simulink model "Quad_Nonlinear_Pitch_PID"  (R2020a)
settings: Solver=ode4  StartTime=0.0  StopTime=15  FixedStep=0.01  RelTol=1e-3
InitFcn:
  | QuadParameter
values from neighbouring files (symbols this model uses):
  AHRS_RCP = AHRS(251:end, :) * pi / 180    [PS_II.m]    (also in RCP_data_I.m; RCP_data_II.m)
  b = 3.13e-5    (= 3.13e-05)    [QuadParameter.m]
  d_cg = 0.2    [QuadParameter.m]
  g = 9.81    [QuadParameter.m]
  h_cg = 0.02    [QuadParameter.m]
  J_yy = 0.03066    [QuadParameter.m]
  KD_Pitch = 10^savedata{1}(3)/15    [RCP_data_I.m]    (also in RCP_data_II.m)
  KI_Pitch = 10^savedata{1}(2)*10    [RCP_data_I.m]    (also in RCP_data_II.m)
  KP_Pitch = 10^savedata{1}(1)/25    [RCP_data_I.m]    (also in RCP_data_II.m)
  m_tot = 0.638    [QuadParameter.m]
undefined symbols (not defined in the file or in its folder): m2, magnitude, miu_k, r_y
libraries: simulink x1
settings Model: OrderedModelArguments=off  Creator=Ali  LastModifiedBy=Ali

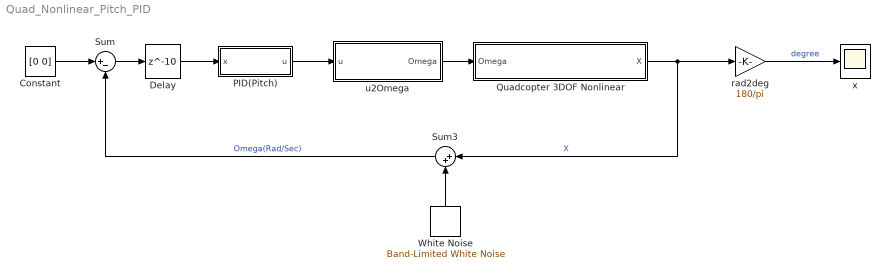
== system Quad_Nonlinear_Pitch_PID ==
  " White Noise" : simulink/Sources/Band-Limited White Noise  Cov=[0.000005]  Ts=.01  seed=[23341]
  Constant : Constant  Value=[0 0]
  Delay : Delay  DelayLength=10
  PID(Pitch) : Subsystem
  Quadcopter 3DOF Nonlinear : Subsystem  TreatAsAtomicUnit=on
  Sum : Sum  Inputs=|+-
  Sum3 : Sum  Inputs=|++
  rad2deg : Gain  Gain=180/pi
  u2Omega : Subsystem
  x : Scope
  wires:
  Quadcopter 3DOF Nonlinear/1(X) -> Sum3/1, rad2deg/1  "X"
  " White Noise"/1 -> Sum3/2
  rad2deg/1 -> x/1  "degree"
  Sum3/1 -> Sum/2  "Omega(Rad/Sec)"
  u2Omega/1(Omega) -> Quadcopter 3DOF Nonlinear/1(Omega)
  Constant/1 -> Sum/1
  PID(Pitch)/1(u) -> u2Omega/1(u)
  Sum/1 -> Delay/1
  Delay/1 -> PID(Pitch)/1(x)

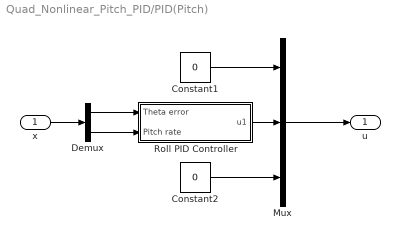
== system Quad_Nonlinear_Pitch_PID/PID(Pitch) ==
  x : Inport
  Constant1 : Constant  Value=0
  Constant2 : Constant  Value=0
  Demux : Demux  Outputs=2
  Mux : Mux  Inputs=3
  Roll PID Controller : Subsystem  VariantControl=Choice
  u : Outport
  wires:
  Mux/1 -> u/1
  x/1 -> Demux/1
  Demux/2 -> Roll PID Controller/2(Pitch rate)
  Constant2/1 -> Mux/3
  Demux/1 -> Roll PID Controller/1(Theta error)
  Roll PID Controller/1(u1) -> Mux/2
  Constant1/1 -> Mux/1

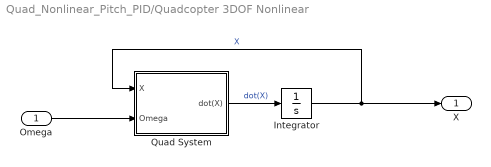
== system Quad_Nonlinear_Pitch_PID/Quadcopter 3DOF Nonlinear ==
  Omega : Inport
  Integrator : Integrator  InitialCondition=AHRS_RCP(1, :)
  Quad System : Subsystem
  X : Outport
  wires:
  Integrator/1 -> Quad System/1(X), X/1  "X"
  Quad System/1(dot(X)) -> Integrator/1  "dot(X)"
  Omega/1 -> Quad System/2(Omega)

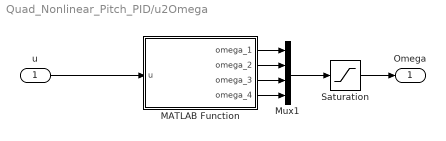
== system Quad_Nonlinear_Pitch_PID/u2Omega ==
  u : Inport
  MATLAB Function : MATLAB Function  TreatAsAtomicUnit=on
  Mux1 : Mux
  Saturation : Saturate  UpperLimit=4000/60*2*pi  LowerLimit=1500/60*2*pi
  Omega : Outport
  wires:
  MATLAB Function/2(omega_2) -> Mux1/2
  u/1 -> MATLAB Function/1(u)
  MATLAB Function/3(omega_3) -> Mux1/3
  MATLAB Function/1(omega_1) -> Mux1/1
  MATLAB Function/4(omega_4) -> Mux1/4
  Mux1/1 -> Saturation/1
  Saturation/1 -> Omega/1

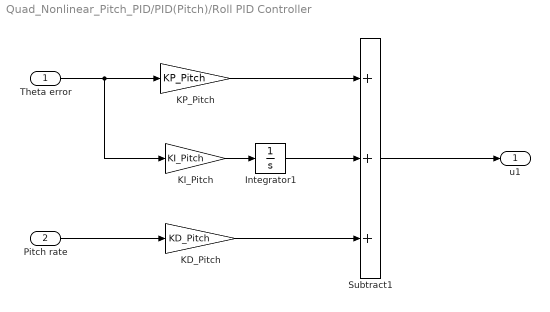
== system Quad_Nonlinear_Pitch_PID/PID(Pitch)/Roll PID Controller ==
  Theta error : Inport
  Pitch rate : Inport  Port=2
  Integrator1 : Integrator
  KD_Pitch : Gain  Gain=KD_Pitch
  KI_Pitch : Gain  Gain=KI_Pitch
  KP_Pitch : Gain  Gain=KP_Pitch
  Subtract1 : Sum  Inputs=+++
  u1 : Outport
  wires:
  Integrator1/1 -> Subtract1/2
  KI_Pitch/1 -> Integrator1/1
  KD_Pitch/1 -> Subtract1/3
  Subtract1/1 -> u1/1
  KP_Pitch/1 -> Subtract1/1
  Pitch rate/1 -> KD_Pitch/1
  Theta error/1 -> KI_Pitch/1, KP_Pitch/1

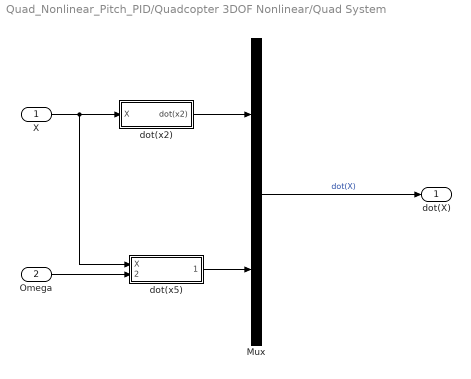
== system Quad_Nonlinear_Pitch_PID/Quadcopter 3DOF Nonlinear/Quad System ==
  X : Inport
  Omega : Inport  Port=2
  Mux : Mux  Inputs=2
  dot(x2) : Subsystem
  dot(x5) : Subsystem
  dot(X) : Outport
  wires:
  Mux/1 -> dot(X)/1  "dot(X)"
  dot(x2)/1(dot(x2)) -> Mux/1
  dot(x5)/1(dot(x5)) -> Mux/2
  X/1 -> dot(x5)/1(X), dot(x2)/1(X)
  Omega/1 -> dot(x5)/2(Omega)

== system Quad_Nonlinear_Pitch_PID/Quadcopter 3DOF Nonlinear/Quad System/dot(x2) ==
  X : Inport
  1 : Subsystem
  dot(x2) : Outport
  wires:
  X/1 -> 1/1(X)  "X"
  1/1(x5cos(x1)) -> dot(x2)/1

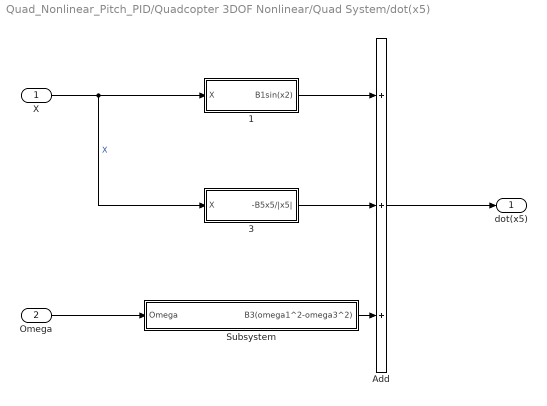
== system Quad_Nonlinear_Pitch_PID/Quadcopter 3DOF Nonlinear/Quad System/dot(x5) ==
  X : Inport
  Omega : Inport  Port=2
  1 : Subsystem
  3 : Subsystem
  Add : Sum  Inputs=+++
  Subsystem : Subsystem
  dot(x5) : Outport
  wires:
  X/1 -> 3/1(X), 1/1(X)  "X"
  Omega/1 -> Subsystem/1(Omega)
  Add/1 -> dot(x5)/1
  Subsystem/1(B3(omega1^2-omega3^2)) -> Add/3
  3/1("-B5x5/|x5| ") -> Add/2
  1/1(B1sin(x2)) -> Add/1

== system Quad_Nonlinear_Pitch_PID/Quadcopter 3DOF Nonlinear/Quad System/dot(x2)/1 ==
  X : Inport
  Selector : Selector  InputPortWidth=2  IndexOptions=Index vector (dialog)  Indices=[2]  OutputSizes=1
  x5cos(x1) : Outport
  wires:
  X/1 -> Selector/1  "x"
  Selector/1 -> x5cos(x1)/1

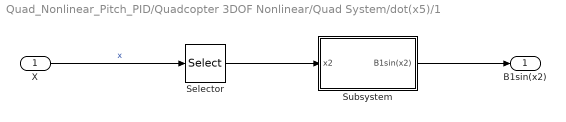
== system Quad_Nonlinear_Pitch_PID/Quadcopter 3DOF Nonlinear/Quad System/dot(x5)/1 ==
  X : Inport
  Selector : Selector  InputPortWidth=2  IndexOptions=Index vector (dialog)  Indices=[1]  OutputSizes=1
  Subsystem : Subsystem
  B1sin(x2) : Outport
  wires:
  X/1 -> Selector/1  "x"
  Subsystem/1(B1sin(x2)) -> B1sin(x2)/1
  Selector/1 -> Subsystem/1(x2)

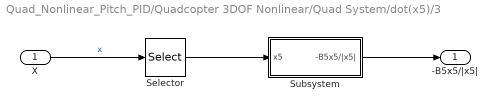
== system Quad_Nonlinear_Pitch_PID/Quadcopter 3DOF Nonlinear/Quad System/dot(x5)/3 ==
  X : Inport
  Selector : Selector  InputPortWidth=2  IndexOptions=Index vector (dialog)  Indices=[2]  OutputSizes=1
  Subsystem : Subsystem
  "-B5x5/|x5| " : Outport
  wires:
  X/1 -> Selector/1  "x"
  Subsystem/1("-B5x5/|x5| ") -> "-B5x5/|x5| "/1
  Selector/1 -> Subsystem/1(x5)

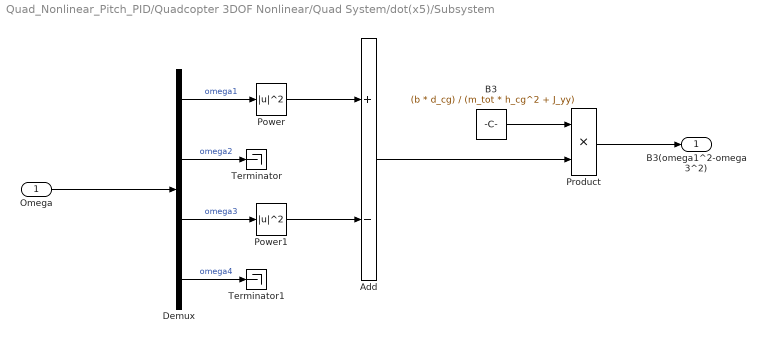
== system Quad_Nonlinear_Pitch_PID/Quadcopter 3DOF Nonlinear/Quad System/dot(x5)/Subsystem ==
  Omega : Inport
  Add : Sum  Inputs=+-
  B3 : Constant  Value=(b * d_cg) / (m_tot * h_cg^2 + J_yy)
  Demux : Demux
  Power : Math  Operator=magnitude^2  SaturateOnIntegerOverflow=on
  Power1 : Math  Operator=magnitude^2  SaturateOnIntegerOverflow=on
  Product : Product
  Terminator : Terminator
  Terminator1 : Terminator
  B3(omega1^2-omega3^2) : Outport
  wires:
  Product/1 -> B3(omega1^2-omega3^2)/1
  Power1/1 -> Add/2
  Add/1 -> Product/2
  Power/1 -> Add/1
  B3/1 -> Product/1
  Omega/1 -> Demux/1
  Demux/3 -> Power1/1  "omega3"
  Demux/1 -> Power/1  "omega1"
  Demux/2 -> Terminator/1  "omega2"
  Demux/4 -> Terminator1/1  "omega4"

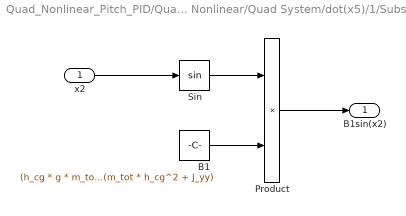
== system Quad_Nonlinear_Pitch_PID/Quadcopter 3DOF Nonlinear/Quad System/dot(x5)/1/Subsystem ==
  x2 : Inport
  B1 : Constant  Value=(h_cg * g * m_tot) / (m_tot * h_cg^2 + J_yy)
  Product : Product
  Sin : Trigonometry
  B1sin(x2) : Outport
  wires:
  Product/1 -> B1sin(x2)/1
  x2/1 -> Sin/1
  B1/1 -> Product/2
  Sin/1 -> Product/1

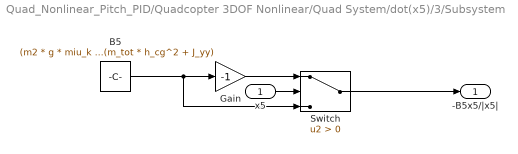
== system Quad_Nonlinear_Pitch_PID/Quadcopter 3DOF Nonlinear/Quad System/dot(x5)/3/Subsystem ==
  x5 : Inport
  B5 : Constant  Value=(m2 * g * miu_k * r_y) / (m_tot * h_cg^2 + J_yy)
  Gain : Gain  Gain=-1
  Switch : Switch  Criteria=u2 > Threshold
  "-B5x5/|x5| " : Outport
  wires:
  Switch/1 -> "-B5x5/|x5| "/1
  B5/1 -> Switch/3, Gain/1
  x5/1 -> Switch/2
  Gain/1 -> Switch/1

== matlab function Quad_Nonlinear_Pitch_PID/u2Omega/MATLAB Function ==
  data: u input size=3; omega_1 output size=1; omega_2 output size=1; omega_3 output size=1; omega_4 output size=1
function [omega_1, omega_2, omega_3, omega_4] = fcn(u)
u1 = u(1);
u2 = u(2);
u3 = u(3);
% control effort
u4 = ones(1, length(u1)) * 4 * rpm2rad_sec(2000)^2;
% calculate omega
if (u4 + u3 + 2 * u2) / 4 > 0
    omega_1 = sqrt((u4 + u3 + 2 * u2) / 4);
else
    omega_1 = 0;
end
if (u4 + u3 - 2 * u2) / 4 > 0
    omega_3 = sqrt((u4 + u3 - 2 * u2) / 4);
else
    omega_3 = 0;
end
if (u4 - u3 + 2 * u1) / 4 > 0
    omega_2 = sqrt((u4 - u3 + 2 * u1) / 4);
else
    omega_2 = 0;
end
if (u4 - u3 - 2 * u1) / 4 > 0
    omega_4 = sqrt((u4 - u3 - 2 * u1) / 4);
else
    omega_4 = 0;
end
end
%% functions
% rpm to rad/sec
function rad = rpm2rad_sec(rpm)
rad = rpm / 60 * 2 * pi;
end
